simulink model "DFIG_LVRT_function_add_20210713_v1"  (R2021a)
settings: Solver=VariableStepAuto  StartTime=0.0  StopTime=4.3  FixedStep=50e-6  RelTol=1e-3
InitFcn:
  | init;
values from neighbouring files (symbols this model uses):
  a11 = -Rs/sigma/Ls    (= -15.198082107)    [init.m]
  a13 = Rs*Lm/sigma/Ls/Lr    (= 14.6869753643)    [init.m]
  a22 = a11    (= -15.198082107)    [init.m]
  a24 = a13    (= 14.6869753643)    [init.m]
  a31 = Rr*Lm/sigma/Ls/Lr    (= 16.3816263679)    [init.m]
  a33 = -Rr/sigma/Ls    (= -16.9517069655)    [init.m]
  a42 = a31    (= 16.3816263679)    [init.m]
  a44 = a33    (= -16.9517069655)    [init.m]
  Cbus = 80e-3    (= 0.08)    [init.m]
  D = 1e-3 * 0    (= 0)    [init.m]
  f = 50    [init.m]
  Fs = Vs * sqrt(2/3)/(2*pi*f)    [init.m]
  fsw = 4e3    (= 4000)    [init.m]
  Is = 1760    [init.m]
  J = 127    [init.m]
  Kopt = ((0.5*ro*pi*(Rayon^5)*Cp_max)/(lambda_opt^3))    (= 296454.198186)    [init.m]
  Kpg = 1/(1.5*Vs*sqrt(2/3))    [init.m]
  Kqg = -Kpg    [init.m]
  Lg = 400e-6    (= 0.0004)    [init.m]
  Lm = 2.5e-3    (= 0.0025)    [init.m]
  Lr = Lm + Lsi    (= 0.002587)    [init.m]
  Ls = Lm + Lsi    (= 0.002587)    [init.m]
  Lsi = 0.087e-3    (= 8.7e-05)    [init.m]
  N = 100    [init.m]
  p = 2    [init.m]
  Ps = 2e6    (= 2000000)    [init.m]
  Rcrowbar = 1/5    (= 0.2)    [init.m]
  Rg = 20e-6    (= 2e-05)    [init.m]
  Rr = 2.9e-3    (= 0.0029)    [init.m]
  Rs = 2.6e-3    (= 0.0026)    [init.m]
  sigma = 1 - Lm^2/(Ls*Lr)    (= 0.0661284179513)    [init.m]
  smax = 1/3    (= 0.333333333333)    [init.m]
  Tem = 12732    [init.m]
  Ts = 1/fsw/50    (= 5e-06)    [init.m]
  Vbus = 1150    [init.m]
  Vs = 690    [init.m]
undefined symbols (not defined in the file or in its folder): DiscIntNeverNeededParam
libraries: DFIM_Tutorial_Library x37, spsSecondOrderFilterLib x8, spsSeriesRLCBranchLib x5, spsThreePhaseVIMeasurementLib x4, spsUniversalBridgeLib x3, spsPLL3phLib x2, spsPWMGenerator2LevelLib x2, spsAsynchronousMachineSIUnitsLib x1, spsGroundLib x1, spsThreePhaseTransformerTwoWindingsLib x1, spsIdealSwitchLib x1, spsMultimeterLib x1
settings Model: SimulationMode=accelerator  Creator=anony  LastModifiedBy=anony
settings SolverCC: AlgebraicLoopSolver=TrustRegion
settings DebuggingCC: UnconnectedInputMsg=none  UnconnectedOutputMsg=none  UnconnectedLineMsg=none  SFMachineParentedDataDiag=warning

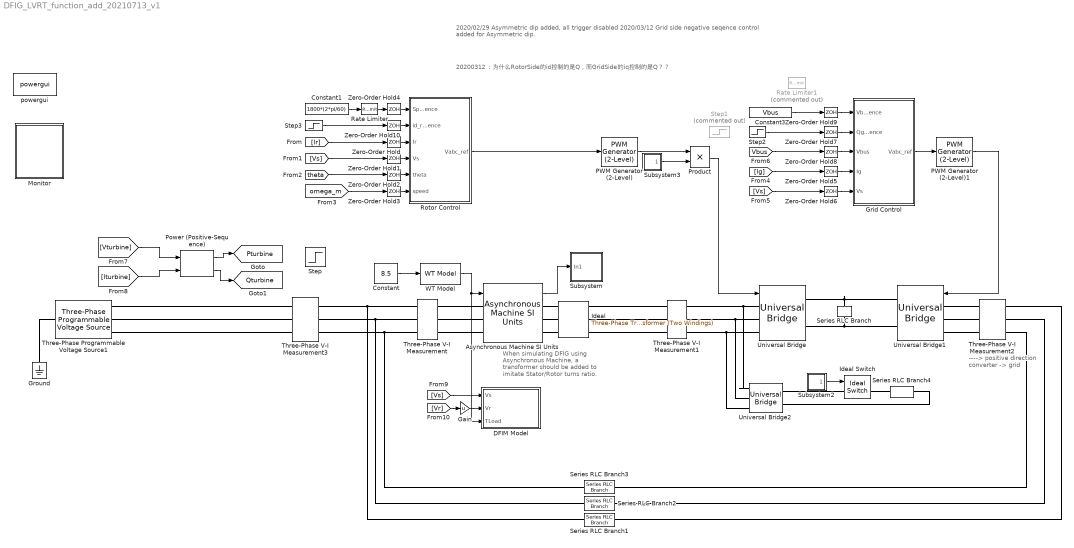
== system DFIG_LVRT_function_add_20210713_v1 ==
  note: 20200312：为什么RotorSide的id控制的是Q，而GridSide的iq控制的是Q？？
  note: ---->
      | positive direction
      | converter -> grid
  note: When simulating DFIG using Asynchronous Machine,
      | a transformer should be added to imitate Stator/Rotor turns
      | ratio.
  note: 2020/02/29 Asymmetric dip added, all trigger disabled
      | 2020/03/12 Grid side negative seqence control added for Asymmetric dip.
  Asynchronous Machine SI Units : spsAsynchronousMachineSIUnitsLib/Asynchronous Machine SI Units  RotorType=Wound  PresetModel=No  MechanicalLoad=Torque Tm  ShowDetailedParameters=on  ReferenceFrame=Rotor  Units=SI  MeasurementBus=off  NominalParameters=[Ps Vs f]  VoltageRatio=1  Stator=[Rs Lsi]  Rotor=[Rr Lsi]  Cage1=[0.4155 0.002066]  Cage2=[0.4168 0.0003495]  Lm=Lm  Mechanical=[J D p]  PolePairs=2  InitialConditions=[1 0 0 0 0 0 0 0]  SimulateSaturation=off  Saturation=[14.03593122, 27.81365428, 53.79336849, 72.68890987, 97.98006896, 148.6815601, 215.7428561, 302.9841135, 428.7778367 ; 230, 322, 414, 460, 506, 552, 598, 644, 690]  LoadFlowParameters=1492000  TsPowergui=0  TsBlock=-1  IterativeModel=Trapezoidal non iterative  IterativeDiscreteModel=Trapezoidal non iterative  Pmec=1.492e+006
  Constant : Constant  Value=8.5
  Constant1 : Constant  Value=1800*(2*pi/60)
  Constant3 : Constant  Value=Vbus
  DFIM Model : Subsystem
  Gain : Gain  Gain=u
  Grid Control : Subsystem
  Ground : spsGroundLib/Ground  LConnTagsString=a
  Ideal : spsThreePhaseTransformerTwoWindingsLib/Three-Phase Transformer (Two Windings)  Winding1Connection=Y  Winding2Connection=Y  CoreType=Three single-phase transformers  SetSaturation=off  Hysteresis=off  DataFile='hysteresis'  SetInitialFlux=off  Measurements=None  UNITS=SI  NominalPower=[ Ps , f ]  Winding1=[Vs 0 0]  Winding2=[Vs/u 0 0]  Rm="1.0805e+06  % keep this at a high value"  Lm="2866  % keep this at a high value"  L0=0.5  Saturation=[0 0;0.66653 1910.3;277.72 2419.7]  InitialFluxes=[ 0.8 , -0.8 , 0.7 ]  BreakLoop=off  DiscreteSolver=Trapezoidal iterative  DataType=on  TransfoNumber=1
  Ideal Switch : spsIdealSwitchLib/Ideal Switch  Ron=0.001  Lon=0  IC=0  Rs=1e5  Cs=inf  Measurements=on
  Monitor : Subsystem
  PWM Generator (2-Level) : spsPWMGenerator2LevelLib/PWM Generator (2-Level)  ModulatorType=Three-phase bridge (6 pulses)  ModulatorMode=Unsynchronized  Fc=fsw  Pc=90  nF=27  MinMax="[ -1  1 ]"  SamplingTechnique=Symmetrical regular (single edge)  ModulatingSignals=off  m=0.8  Freq=60  Phase=0  Ts=0  ShowCarrierOutport=off
  PWM Generator (2-Level)1 : spsPWMGenerator2LevelLib/PWM Generator (2-Level)  ModulatorType=Three-phase bridge (6 pulses)  ModulatorMode=Unsynchronized  Fc=fsw  Pc=0  nF=27  MinMax="[ -1  1 ]"  SamplingTechnique=Symmetrical regular (single edge)  ModulatingSignals=off  m=0.8  Freq=60  Phase=0  Ts=0  ShowCarrierOutport=off
  Power (Positive-Sequence) : spsPowerPositiveSequenceLib/Power (Positive-Sequence)  Freq=50  Vinit=[0, 0]  Iinit=[0, 0]  Ts=0
      settings: SourceProductBaseCode=PS
  Product : Product
  Rate Limiter : RateLimiter  RisingSlewLimit=100/1  FallingSlewLimit=-100/1  SampleTimeMode=inherited
  Rate Limiter1 : RateLimiter  Commented=on  RisingSlewLimit=1000e3/2  FallingSlewLimit=-1000e3/2  SampleTimeMode=inherited
  Rotor Control : Subsystem
  Series RLC Branch : spsSeriesRLCBranchLib/Series RLC Branch  LConnTagsString=__new0  RConnTagsString=__new0  BranchType=C  Resistance=1  Inductance=1e-3  SetiL0=off  InitialCurrent=0  Capacitance=Cbus  Setx0=on  InitialVoltage=0  Measurements=Branch voltage
  Series RLC Branch1 : spsSeriesRLCBranchLib/Series RLC Branch  LConnTagsString=__new0  RConnTagsString=__new0  BranchType=RL  Resistance=Rg  Inductance=Lg  SetiL0=off  InitialCurrent=0  Capacitance=Cbus  Setx0=on  InitialVoltage=0  Measurements=None
  Series RLC Branch2 : spsSeriesRLCBranchLib/Series RLC Branch  LConnTagsString=__new0  RConnTagsString=__new0  BranchType=RL  Resistance=Rg  Inductance=Lg  SetiL0=off  InitialCurrent=0  Capacitance=Cbus  Setx0=on  InitialVoltage=0  Measurements=None
  Series RLC Branch3 : spsSeriesRLCBranchLib/Series RLC Branch  LConnTagsString=__new0  RConnTagsString=__new0  BranchType=RL  Resistance=Rg  Inductance=Lg  SetiL0=off  InitialCurrent=0  Capacitance=Cbus  Setx0=on  InitialVoltage=0  Measurements=None
  Series RLC Branch4 : spsSeriesRLCBranchLib/Series RLC Branch  LConnTagsString=__new0  RConnTagsString=__new0  BranchType=R  Resistance=Rcrowbar  Inductance=1e-3  SetiL0=off  InitialCurrent=0  Capacitance=Cbus  Setx0=on  InitialVoltage=0  Measurements=Branch current
  Step : Step  Time=3.453  Before=7.5  After=11  SampleTime=0
  Step1 : Step  Commented=on  Time=4.084  After=-400e3  SampleTime=0
  Step2 : Step  Time=3.15  After=-500e3  SampleTime=0
  Step3 : Step  Time=3.15  After=Is*0.25  SampleTime=0
  Subsystem : Subsystem
  Subsystem2 : Subsystem
  Subsystem3 : Subsystem
  Three-Phase Programmable Voltage Source1 : spsThreePhaseProgrammableVoltageSourceLib/Three-Phase Programmable Voltage Source  PositiveSequence=[Vs 0 f]  VariationEntity=None  VariationType=Ramp  VariationTypeAlt=Step  VariationStep=0.5  VariationRate=15  VariationMagnitude=0.3  VariationFrequency=2  VariationTiming=[3.5 4.17]  VariationPhaseA=off  Amplitudes=[1 0.8 1.2 1.0]  TimeValues=[0 0.1 0.15 0.2]  HarmonicGeneration=on  HarmonicA=[1 0.3 180 1]  HarmonicB=[1 0.2 0 2]  Timing="[3  4.2]"  BusType=swing  Pref=0  Qref=0  Qmin=-inf  Qmax=inf
  Three-Phase V-I Measurement : spsThreePhaseVIMeasurementLib/Three-Phase V-I Measurement  VoltageMeasurement=phase-to-ground  SetLabelV=on  LabelV=Vs  Vpu=off  VpuLL=off  CurrentMeasurement=yes  SetLabelI=on  LabelI=Is  Ipu=off  Pbase=100e6  Vbase=500e3  OutputType=Complex  PhasorSimulation=off  PSBequivalent=0
  Three-Phase V-I Measurement1 : spsThreePhaseVIMeasurementLib/Three-Phase V-I Measurement  VoltageMeasurement=phase-to-ground  SetLabelV=on  LabelV=Vr  Vpu=off  VpuLL=off  CurrentMeasurement=yes  SetLabelI=on  LabelI=Ir  Ipu=off  Pbase=100e6  Vbase=500e3  OutputType=Complex  PhasorSimulation=off  PSBequivalent=0
  Three-Phase V-I Measurement2 : spsThreePhaseVIMeasurementLib/Three-Phase V-I Measurement  VoltageMeasurement=no  SetLabelV=on  LabelV=Vs  Vpu=on  VpuLL=off  CurrentMeasurement=yes  SetLabelI=on  LabelI=Ig  Ipu=off  Pbase=100e6  Vbase=500e3  OutputType=Complex  PhasorSimulation=off  PSBequivalent=0
  Three-Phase V-I Measurement3 : spsThreePhaseVIMeasurementLib/Three-Phase V-I Measurement  VoltageMeasurement=phase-to-ground  SetLabelV=on  LabelV=Vturbine  Vpu=off  VpuLL=off  CurrentMeasurement=yes  SetLabelI=on  LabelI=Iturbine  Ipu=off  Pbase=100e6  Vbase=500e3  OutputType=Complex  PhasorSimulation=off  PSBequivalent=0
  Universal Bridge : spsUniversalBridgeLib/Universal Bridge  Arms=3  SnubberResistance=1e5  SnubberCapacitance=inf  Device=Ideal Switches  Ron=1e-3  Lon=0  ForwardVoltages="[  0  0  ]"  ForwardVoltage=0  GTOparameters=[ 10e-6 , 20e-6 ]  IGBTparameters=[ 1e-6 , 2e-6 ]  Measurements=None  Measurements_2=None  converterType=Rectifier
  Universal Bridge1 : spsUniversalBridgeLib/Universal Bridge  Arms=3  SnubberResistance=1e5  SnubberCapacitance=inf  Device=Ideal Switches  Ron=1e-3  Lon=0  ForwardVoltages="[  0  0  ]"  ForwardVoltage=0  GTOparameters=[ 10e-6 , 20e-6 ]  IGBTparameters=[ 1e-6 , 2e-6 ]  Measurements=None  Measurements_2=None  converterType=Rectifier
  Universal Bridge2 : spsUniversalBridgeLib/Universal Bridge  Arms=3  SnubberResistance=1e5  SnubberCapacitance=inf  Device=Diodes  Ron=1e-3  Lon=0  ForwardVoltages="[  0  0  ]"  ForwardVoltage=0  GTOparameters=[ 10e-6 , 20e-6 ]  IGBTparameters=[ 1e-6 , 2e-6 ]  Measurements=None  Measurements_2=None  converterType=Rectifier
  WT Model : DFIM_Tutorial_Library/WT Model  SystemSampleTime=-1  VariantActivationTime=update diagram  Latency=0  AutoFrameSizeCalculation=off
  Zero-Order Hold{,1..10} (11 alike) : ZeroOrderHold  SampleTime=1/fsw
  powergui : spspowerguiLib/powergui  Priority=1  SimulationMode=Discrete  SampleTime=Ts  frequency=60  Iterations=50  frequencyindice=50  Pbase=100e6  ErrMax=1e-4  UnitsV=kV  UnitsW=MW  buscounter=0  FunctionMessages=off  echomessages=off  EnableUseOfTLC=off  CurrentSourceSwitches=off  DisableSnubberDevices=off  DisableRonSwitches=off  DisableVfSwitches=off  DisplayEquations=off  AutomaticDiscreteSolvers=off  SolverType=Tustin/Backward Euler (TBE)  Interpol=off  ExternalGateDelay=off  methode=off  Ts=100  x0status=blocks  SPID=on  SwTol=0  HookPort=off  NonlinearTolerance=1e-4  nMaxIteration=100  ContinueOnMaxIteration=off  RestoreLinks=warning  ResistiveCurrentMeasurement=off  Frange=[0:2:500]  Ylog=off  Xlog=on  ShowGrid=off  save=off  variable=ZData  structure=0  ZoomFFT=off  StartTime=0.0  cycles=1  DisplayStyle=1  fundamental=60  FreqAxis=off  MaxFrequency=1000  frequencyindicesteady=1  RmsSteady=1  display=off
  tag scope: Pturbine=global, Qturbine=global
  wires:
  Rotor Control/1(Vabc_ref) -> PWM Generator (2-Level)/1
  [Ir] -> Zero-Order Hold/1
  [Vs] -> Zero-Order Hold1/1
  Asynchronous Machine SI Units/1 -> Subsystem/1(In1)
  [theta] -> Zero-Order Hold2/1
  [omega_m] -> Zero-Order Hold3/1
  Step3/1 -> Zero-Order Hold10/1
  Zero-Order Hold/1 -> Rotor Control/3(Ir)
  Zero-Order Hold1/1 -> Rotor Control/4(Vs)
  Zero-Order Hold2/1 -> Rotor Control/5(theta)
  Zero-Order Hold3/1 -> Rotor Control/6(speed)
  Constant1/1 -> Rate Limiter/1
  Rate Limiter/1 -> Zero-Order Hold4/1
  Zero-Order Hold4/1 -> Rotor Control/1(Speed reference)
  WT Model/1 -> DFIM Model/3(TLoad), Asynchronous Machine SI Units/1
  PWM Generator (2-Level)1/1 -> Universal Bridge1/1
  Zero-Order Hold5/1 -> Grid Control/4(Ig)
  [Vs] -> Zero-Order Hold6/1
  Zero-Order Hold6/1 -> Grid Control/5(Vs)
  [Ig] -> Zero-Order Hold5/1
  Zero-Order Hold9/1 -> Grid Control/1(Vbus reference)
  Constant3/1 -> Zero-Order Hold9/1
  Grid Control/1(Vabc_ref) -> PWM Generator (2-Level)1/1
  Step2/1 -> Zero-Order Hold7/1
  Zero-Order Hold7/1 -> Grid Control/2(Qg_reference)
  [Vbus] -> Zero-Order Hold8/1
  Zero-Order Hold8/1 -> Grid Control/3(Vbus)
  Subsystem2/1(Trig) -> Ideal Switch/1
  Zero-Order Hold10/1 -> Rotor Control/2(id_reference)
  Subsystem3/1(Trig) -> Product/2
  PWM Generator (2-Level)/1 -> Product/1
  Product/1 -> Universal Bridge/1
  Constant/1 -> WT Model/1
  [Vturbine] -> Power (Positive-Sequence)/1
  [Iturbine] -> Power (Positive-Sequence)/2
  Power (Positive-Sequence)/2 -> [Qturbine]
  Power (Positive-Sequence)/1 -> [Pturbine]
  [Vs] -> DFIM Model/1(Vs)
  [Vr] -> Gain/1
  Gain/1 -> DFIM Model/2(Vr)
  connections:
  Three-Phase Programmable Voltage Source1/LConn1 -- Ground/LConn1
  Three-Phase V-I Measurement1/LConn1 -- Universal Bridge2/LConn1 -- Universal Bridge/LConn1
  Three-Phase V-I Measurement1/LConn2 -- Universal Bridge2/LConn2 -- Universal Bridge/LConn2
  Three-Phase V-I Measurement1/LConn3 -- Universal Bridge2/LConn3 -- Universal Bridge/LConn3
  Series RLC Branch1/RConn1 -- Three-Phase V-I Measurement3/LConn1 -- Three-Phase V-I Measurement/LConn1
  Series RLC Branch2/RConn1 -- Three-Phase V-I Measurement/LConn2 -- Three-Phase V-I Measurement3/LConn2
  Series RLC Branch3/RConn1 -- Three-Phase V-I Measurement3/LConn3 -- Three-Phase V-I Measurement/LConn3
  Three-Phase V-I Measurement/RConn1 -- Asynchronous Machine SI Units/LConn1
  Three-Phase V-I Measurement/RConn2 -- Asynchronous Machine SI Units/LConn2
  Three-Phase V-I Measurement/RConn3 -- Asynchronous Machine SI Units/LConn3
  Universal Bridge/RConn1 -- Series RLC Branch/LConn1 -- Universal Bridge1/RConn1
  Universal Bridge/RConn2 -- Series RLC Branch/RConn1 -- Universal Bridge1/RConn2
  Three-Phase V-I Measurement2/LConn1 -- Universal Bridge1/LConn1
  Three-Phase V-I Measurement2/LConn2 -- Universal Bridge1/LConn2
  Three-Phase V-I Measurement2/LConn3 -- Universal Bridge1/LConn3
  Series RLC Branch1/LConn1 -- Three-Phase V-I Measurement2/RConn1
  Three-Phase V-I Measurement2/RConn2 -- Series RLC Branch2/LConn1
  Series RLC Branch3/LConn1 -- Three-Phase V-I Measurement2/RConn3
  Ideal/LConn1 -- Asynchronous Machine SI Units/RConn1
  Ideal/LConn2 -- Asynchronous Machine SI Units/RConn2
  Ideal/LConn3 -- Asynchronous Machine SI Units/RConn3
  Ideal/RConn1 -- Three-Phase V-I Measurement1/RConn1
  Ideal/RConn2 -- Three-Phase V-I Measurement1/RConn2
  Ideal/RConn3 -- Three-Phase V-I Measurement1/RConn3
  Series RLC Branch4/LConn1 -- Ideal Switch/RConn1
  Series RLC Branch4/RConn1 -- Universal Bridge2/RConn2
  Universal Bridge2/RConn1 -- Ideal Switch/LConn1
  Three-Phase Programmable Voltage Source1/RConn1 -- Three-Phase V-I Measurement3/RConn1
  Three-Phase Programmable Voltage Source1/RConn2 -- Three-Phase V-I Measurement3/RConn2
  Three-Phase Programmable Voltage Source1/RConn3 -- Three-Phase V-I Measurement3/RConn3

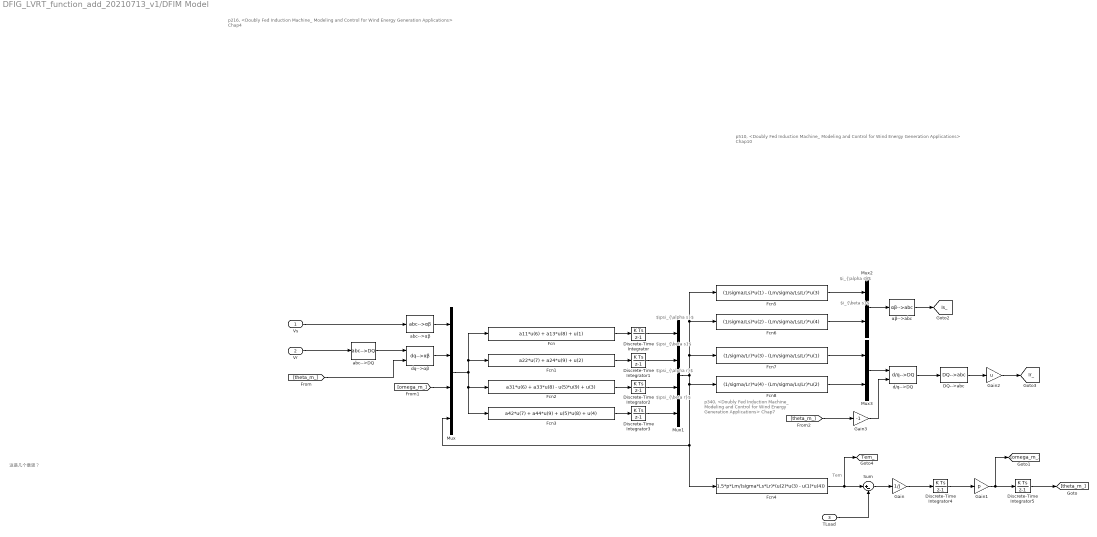
== system DFIG_LVRT_function_add_20210713_v1/DFIM Model ==
  note: p340, <Doubly Fed Induction Machine_ Modeling and Control for Wind Energy Generation Applications> Chap7
  note: $\psi_{\alpha s}$
  note: p510, <Doubly Fed Induction Machine_ Modeling and Control for Wind Energy Generation Applications> Chap10
  note: 这是几个意思？
  note: Tem
  note: p216, <Doubly Fed Induction Machine_ Modeling and Control for Wind Energy Generation Applications> Chap4
  note: $\psi_{\beta s}$
  note: $\psi_{\alpha r}$
  note: $\psi_{\beta r}$
  note: $i_{\alpha s}$
  note: $i_{\beta s}$
  Vs : Inport
  Vr : Inport  Port=2
  TLoad : Inport  Port=3
  DQ-->abc : DFIM_Tutorial_Library/DQ-->abc  SystemSampleTime=-1  VariantActivationTime=update diagram  Latency=0  AutoFrameSizeCalculation=off
  Discrete-Time Integrator{,1..5} (6 alike) : DiscreteIntegrator  SampleTime=Ts  UpperSaturationLimit=1  LowerSaturationLimit=-1  ICPrevOutput=DiscIntNeverNeededParam  ICPrevScaledInput=DiscIntNeverNeededParam
  Fcn : Fcn  Expr=a11*u(6) + a13*u(8) + u(1)
  Fcn1 : Fcn  Expr=a22*u(7) + a24*u(9) + u(2)
  Fcn2 : Fcn  Expr=a31*u(6) + a33*u(8) - u(5)*u(9) + u(3)
  Fcn3 : Fcn  Expr=a42*u(7) + a44*u(9) + u(5)*u(8) + u(4)
  Fcn4 : Fcn  Expr=1.5*p*Lm/(sigma*Ls*Lr)*(u(2)*u(3) - u(1)*u(4))
  Fcn5 : Fcn  Expr=(1/sigma/Ls)*u(1) - (Lm/sigma/Ls/Lr)*u(3)
  Fcn6 : Fcn  Expr=(1/sigma/Ls)*u(2) - (Lm/sigma/Ls/Lr)*u(4)
  Fcn7 : Fcn  Expr=(1/sigma/Lr)*u(3) - (Lm/sigma/Ls/Lr)*u(1)
  Fcn8 : Fcn  Expr=(1/sigma/Lr)*u(4) - (Lm/sigma/Ls/Lr)*u(2)
  Gain : Gain  Gain=1/J
  Gain1 : Gain  Gain=p
  Gain2 : Gain  Gain=u
  Gain3 : Gain  Gain=-1
  Mux : Mux
  Mux1 : Mux
  Mux2 : Mux  Inputs=2
  Mux3 : Mux  Inputs=2
  Sum : Sum  Inputs=|+-
  abc-->DQ : DFIM_Tutorial_Library/abc-->DQ  SystemSampleTime=-1  VariantActivationTime=update diagram  Latency=0  AutoFrameSizeCalculation=off
  abc-->αβ : DFIM_Tutorial_Library/abc-->αβ  SystemSampleTime=-1  VariantActivationTime=update diagram  Latency=0  AutoFrameSizeCalculation=off
  d/q-->DQ : DFIM_Tutorial_Library/d//q-->DQ  SystemSampleTime=-1  VariantActivationTime=update diagram  Latency=0  AutoFrameSizeCalculation=off
  dq-->αβ : DFIM_Tutorial_Library/dq-->αβ  SystemSampleTime=-1  VariantActivationTime=update diagram  Latency=0  AutoFrameSizeCalculation=off
  αβ-->abc : DFIM_Tutorial_Library/αβ-->abc  SystemSampleTime=-1  VariantActivationTime=update diagram  Latency=0  AutoFrameSizeCalculation=off
  tag scope: Ir_=global, Is_=global, Tem_=global
  wires:
  Mux/1 -> Fcn3/1, Fcn2/1, Fcn1/1, Fcn/1
  Fcn/1 -> Discrete-Time Integrator/1
  Fcn1/1 -> Discrete-Time Integrator1/1
  Fcn2/1 -> Discrete-Time Integrator2/1
  Fcn3/1 -> Discrete-Time Integrator3/1
  Discrete-Time Integrator1/1 -> Mux1/2
  Discrete-Time Integrator/1 -> Mux1/1
  Discrete-Time Integrator2/1 -> Mux1/3
  Discrete-Time Integrator3/1 -> Mux1/4
  Mux1/1 -> Fcn7/1, Fcn6/1, Fcn5/1, Mux/4, Fcn4/1, Fcn8/1
  Gain/1 -> Discrete-Time Integrator4/1
  Discrete-Time Integrator4/1 -> Gain1/1
  Gain1/1 -> [omega_m_], Discrete-Time Integrator5/1
  Discrete-Time Integrator5/1 -> [theta_m_]
  Sum/1 -> Gain/1
  Fcn4/1 -> [Tem_], Sum/1
  Vs/1 -> abc-->αβ/1
  abc-->αβ/1 -> Mux/1
  abc-->DQ/1 -> dq-->αβ/1
  dq-->αβ/1 -> Mux/2
  [theta_m_] -> dq-->αβ/2
  Vr/1 -> abc-->DQ/1
  [omega_m_] -> Mux/3
  TLoad/1 -> Sum/2
  Fcn6/1 -> Mux2/2
  Fcn5/1 -> Mux2/1
  Mux2/1 -> αβ-->abc/1
  αβ-->abc/1 -> [Is_]
  DQ-->abc/1 -> Gain2/1
  d/q-->DQ/1 -> DQ-->abc/1
  Fcn7/1 -> Mux3/1
  Fcn8/1 -> Mux3/2
  Gain3/1 -> d/q-->DQ/2
  Mux3/1 -> d/q-->DQ/1
  [theta_m_] -> Gain3/1
  Gain2/1 -> [Ir_]

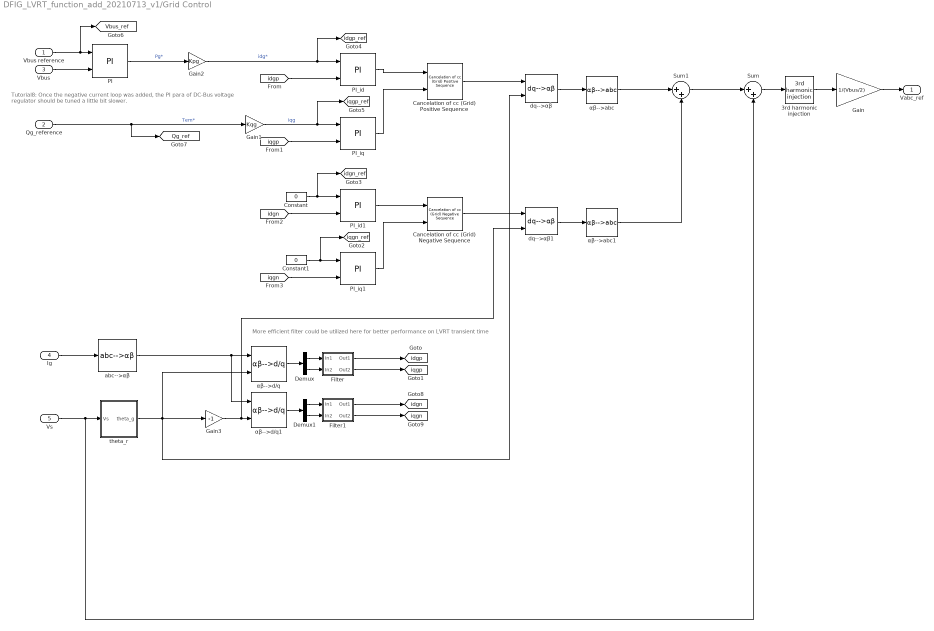
== system DFIG_LVRT_function_add_20210713_v1/Grid Control ==
  note: More efficient filter could be utilized here for better performance on LVRT transient time
  note: Tutorial8: Once the negative current loop was added, the PI para of DC-Bus voltage
      | regulator should be tuned a little bit slower.
  Vbus reference : Inport
  Qg_reference : Inport  Port=2
  Vbus : Inport  Port=3
  Ig : Inport  Port=4
  Vs : Inport  Port=5
  3rd harmonic injection : DFIM_Tutorial_Library/3rd harmonic injection  SystemSampleTime=-1  VariantActivationTime=update diagram  Latency=0  AutoFrameSizeCalculation=off
  Cancelation of cc (Grid) Negative Sequence : DFIM_Tutorial_Library/Cancelation of cc (Grid) Negative Sequence  SystemSampleTime=-1  VariantActivationTime=update diagram  Latency=0  AutoFrameSizeCalculation=off
  Cancelation of cc (Grid) Positive Sequence : DFIM_Tutorial_Library/Cancelation of cc (Grid) Positive Sequence  SystemSampleTime=-1  VariantActivationTime=update diagram  Latency=0  AutoFrameSizeCalculation=off
  Constant : Constant  Value=0
  Constant1 : Constant  Value=0
  Demux : Demux  Outputs=2
  Demux1 : Demux  Outputs=2
  Filter : Subsystem
  Filter1 : Subsystem
  Gain : Gain  Gain=1/(Vbus/2)
  Gain1 : Gain  Gain=Kqg
  Gain2 : Gain  Gain=Kpg
  Gain3 : Gain  Gain=-1
  PI : DFIM_Tutorial_Library/PI  kp=kp_v  ki=ki_v  int_uppper_limit=Ps*smax  int_lower_limit=-Ps*smax  total_upper_limit=Ps*smax  total_lower_limit=-Ps*smax  sample_time=1/fsw
  PI_id : DFIM_Tutorial_Library/PI  kp=kp_idg  ki=ki_idg  int_uppper_limit=Vbus/sqrt(3)  int_lower_limit=-Vbus/sqrt(3)  total_upper_limit=Vbus/sqrt(3)  total_lower_limit=-Vbus/sqrt(3)  sample_time=1/fsw
  PI_id1 : DFIM_Tutorial_Library/PI  kp=kp_idg  ki=ki_idg  int_uppper_limit=Vbus/sqrt(3)  int_lower_limit=-Vbus/sqrt(3)  total_upper_limit=Vbus/sqrt(3)  total_lower_limit=-Vbus/sqrt(3)  sample_time=1/fsw
  PI_iq : DFIM_Tutorial_Library/PI  kp=kp_iqg  ki=ki_iqg  int_uppper_limit=Vbus/sqrt(3)  int_lower_limit=-Vbus/sqrt(3)  total_upper_limit=Vbus/sqrt(3)  total_lower_limit=-Vbus/sqrt(3)  sample_time=1/fsw
  PI_iq1 : DFIM_Tutorial_Library/PI  kp=kp_iqg  ki=ki_iqg  int_uppper_limit=Vbus/sqrt(3)  int_lower_limit=-Vbus/sqrt(3)  total_upper_limit=Vbus/sqrt(3)  total_lower_limit=-Vbus/sqrt(3)  sample_time=1/fsw
  Sum : Sum  Inputs=|++
  Sum1 : Sum  Inputs=|++
  abc-->αβ : DFIM_Tutorial_Library/abc-->αβ  SystemSampleTime=-1  VariantActivationTime=update diagram  Latency=0  AutoFrameSizeCalculation=off
  dq-->αβ : DFIM_Tutorial_Library/dq-->αβ  SystemSampleTime=-1  VariantActivationTime=update diagram  Latency=0  AutoFrameSizeCalculation=off
  dq-->αβ1 : DFIM_Tutorial_Library/dq-->αβ  SystemSampleTime=-1  VariantActivationTime=update diagram  Latency=0  AutoFrameSizeCalculation=off
  theta_r : Subsystem
  αβ-->abc : DFIM_Tutorial_Library/αβ-->abc  SystemSampleTime=-1  VariantActivationTime=update diagram  Latency=0  AutoFrameSizeCalculation=off
  αβ-->abc1 : DFIM_Tutorial_Library/αβ-->abc  SystemSampleTime=-1  VariantActivationTime=update diagram  Latency=0  AutoFrameSizeCalculation=off
  αβ-->d/q : DFIM_Tutorial_Library/αβ-->d//q  SystemSampleTime=-1  VariantActivationTime=update diagram  Latency=0  AutoFrameSizeCalculation=off
  αβ-->d/q1 : DFIM_Tutorial_Library/αβ-->d//q  SystemSampleTime=-1  VariantActivationTime=update diagram  Latency=0  AutoFrameSizeCalculation=off
  Vabc_ref : Outport
  tag scope: Qg_ref=global, Vbus_ref=global, idgn=global, idgn_ref=global, idgp=global, idgp_ref=global, iqgn=global, iqgn_ref=global, iqgp=global, iqgp_ref=global
  wires:
  Gain/1 -> Vabc_ref/1
  dq-->αβ/1 -> αβ-->abc/1
  abc-->αβ/1 -> αβ-->d/q1/1, αβ-->d/q/1
  Ig/1 -> abc-->αβ/1
  3rd harmonic injection/1 -> Gain/1
  Vs/1 -> Sum/2, theta_r/1(Vs)
  theta_r/1(theta_g) -> αβ-->d/q/2, dq-->αβ/2, Gain3/1
  PI_id/1 -> Cancelation of cc (Grid) Positive Sequence/1
  Cancelation of cc (Grid) Positive Sequence/1 -> dq-->αβ/1
  PI_iq/1 -> Cancelation of cc (Grid) Positive Sequence/2
  αβ-->d/q/1 -> Demux/1
  Vbus reference/1 -> [Vbus_ref], PI/1
  Gain1/1 -> [iqgp_ref], PI_iq/1  "iqg"
  Qg_reference/1 -> [Qg_ref], Gain1/1  "Tem*"
  PI/1 -> Gain2/1  "Pg*"
  Gain2/1 -> [idgp_ref], PI_id/1  "idg*"
  Vbus/1 -> PI/2
  Sum/1 -> 3rd harmonic injection/1
  dq-->αβ1/1 -> αβ-->abc1/1
  PI_id1/1 -> Cancelation of cc (Grid) Negative Sequence/1
  Cancelation of cc (Grid) Negative Sequence/1 -> dq-->αβ1/1
  PI_iq1/1 -> Cancelation of cc (Grid) Negative Sequence/2
  αβ-->abc/1 -> Sum1/1
  Sum1/1 -> Sum/1
  αβ-->abc1/1 -> Sum1/2
  Constant/1 -> [idgn_ref], PI_id1/1
  Constant1/1 -> [iqgn_ref], PI_iq1/1
  Demux/1 -> Filter/1(In1)
  Demux/2 -> Filter/2(In2)
  Filter/1(Out1) -> [idgp]
  Filter/2(Out2) -> [iqgp]
  Filter1/2(Out2) -> [iqgn]
  Filter1/1(Out1) -> [idgn]
  Demux1/2 -> Filter1/2(In2)
  Demux1/1 -> Filter1/1(In1)
  αβ-->d/q1/1 -> Demux1/1
  Gain3/1 -> dq-->αβ1/2, αβ-->d/q1/2
  [idgp] -> PI_id/2
  [iqgp] -> PI_iq/2
  [iqgn] -> PI_iq1/2
  [idgn] -> PI_id1/2

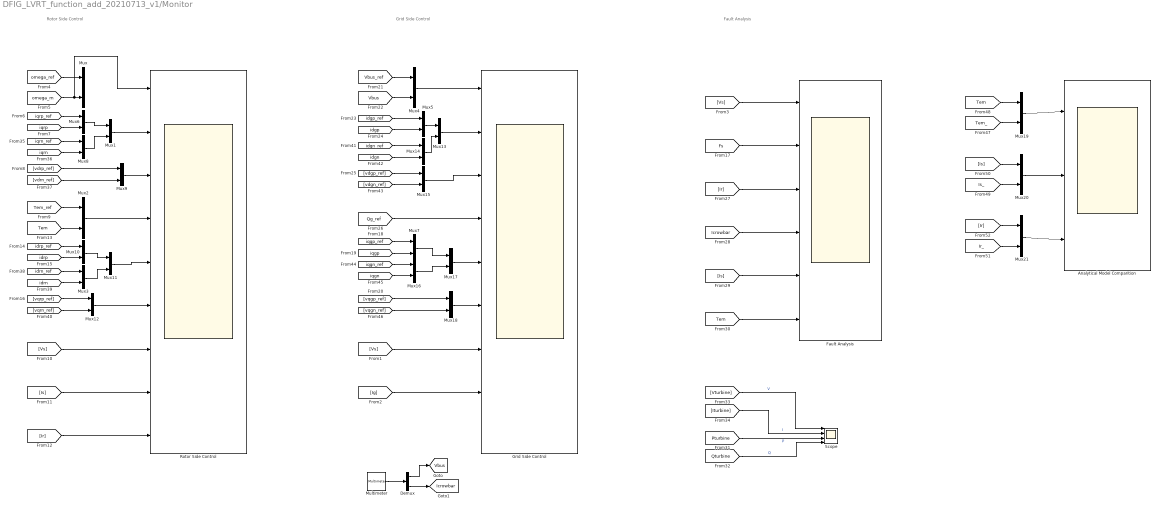
== system DFIG_LVRT_function_add_20210713_v1/Monitor ==
  note: Rotor Side Control
  note: Grid Side Control
  note: Fault Analysis
  Analytical Model Comparition : Scope  NumInputPorts=3
  Demux : Demux  Outputs=2
  Fault Analysis : Scope  NumInputPorts=6
  Grid Side Control : Scope  NumInputPorts=9
  Multimeter : spsMultimeterLib/Multimeter  PhasorSimulation=off  OutputType=Complex  sel=[1 2]  L=2  Gain=[1 1]  yselected={'Ub: Series RLC Branch','Ib: Series RLC Branch4'};  PSBOutputType=1  PSBequivalent=0  AxesSetting=[0,0.1,-100,100]  Display=0  SavedBlockNames=-11
  Mux{,1..21} (22 alike) : Mux  Inputs=2
  Rotor Side Control : Scope  NumInputPorts=9
  Scope : Scope  NumInputPorts=4
  tag scope: Icrowbar=global, Vbus=global
  wires:
  [Tem_ref] -> Mux2/1
  [Ir] -> Rotor Side Control/9
  [Vs] -> Rotor Side Control/7
  [iqrp_ref] -> Mux6/1
  [Tem] -> Mux2/2
  [iqrp] -> Mux6/2
  Mux2/1 -> Rotor Side Control/4
  [Is] -> Rotor Side Control/8
  [omega_m] -> Rotor Side Control/1, Mux/2
  [omega_ref] -> Mux/1
  [Vbus_ref] -> Mux4/1
  [Vbus] -> Mux4/2
  [iqgp_ref] -> Mux7/1
  [Ig] -> Grid Side Control/8
  [idgp] -> Mux5/2
  [iqgp] -> Mux7/2
  [idgp_ref] -> Mux5/1
  [Vs] -> Grid Side Control/7
  [Qg_ref] -> Grid Side Control/4
  Mux4/1 -> Grid Side Control/1
  Multimeter/1 -> Demux/1
  Demux/1 -> [Vbus]
  Demux/2 -> [Icrowbar]
  [Vs] -> Fault Analysis/1
  [Fs] -> Fault Analysis/2
  [Ir] -> Fault Analysis/3
  [Icrowbar] -> Fault Analysis/4
  [Is] -> Fault Analysis/5
  [Tem] -> Fault Analysis/6
  [Pturbine] -> Scope/3  "P"
  [Qturbine] -> Scope/4  "Q"
  [Iturbine] -> Scope/2  "I"
  [Vturbine] -> Scope/1  "V"
  [iqrn_ref] -> Mux8/1
  [iqrn] -> Mux8/2
  Mux6/1 -> Mux1/1
  Mux8/1 -> Mux1/2
  Mux1/1 -> Rotor Side Control/2
  Mux9/1 -> Rotor Side Control/3
  [vdrp_ref] -> Mux9/1
  [vdrn_ref] -> Mux9/2
  [idrp_ref] -> Mux10/1
  [idrp] -> Mux10/2
  [idrn_ref] -> Mux3/1
  [idrn] -> Mux3/2
  Mux10/1 -> Mux11/1
  Mux3/1 -> Mux11/2
  Mux11/1 -> Rotor Side Control/5
  Mux12/1 -> Rotor Side Control/6
  [vqrp_ref] -> Mux12/1
  [vqrn_ref] -> Mux12/2
  Mux13/1 -> Grid Side Control/2
  Mux5/1 -> Mux13/1
  [idgn_ref] -> Mux14/1
  [idgn] -> Mux14/2
  Mux14/1 -> Mux13/2
  Mux15/1 -> Grid Side Control/3
  [vdgp_ref] -> Mux15/1
  [vdgn_ref] -> Mux15/2
  [iqgn] -> Mux16/2
  [iqgn_ref] -> Mux16/1
  Mux17/1 -> Grid Side Control/5
  Mux7/1 -> Mux17/1
  Mux16/1 -> Mux17/2
  Mux18/1 -> Grid Side Control/6
  [vqgp_ref] -> Mux18/1
  [vqgn_ref] -> Mux18/2
  [Tem] -> Mux19/1
  [Tem_] -> Mux19/2
  [Is_] -> Mux20/2
  [Is] -> Mux20/1
  [Ir] -> Mux21/1
  [Ir_] -> Mux21/2
  Mux19/1 -> Analytical Model Comparition/1
  Mux20/1 -> Analytical Model Comparition/2
  Mux21/1 -> Analytical Model Comparition/3

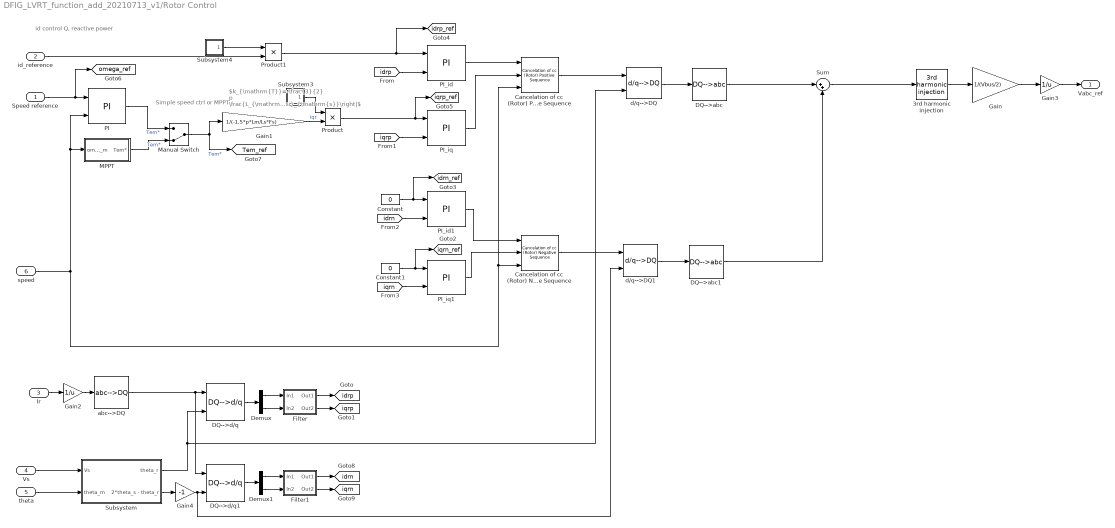
== system DFIG_LVRT_function_add_20210713_v1/Rotor Control ==
  note: id control Q, reactive power
  note: Simple speed ctrl
      | or MPPT
  note: $k_{\mathrm{T}}=-\frac{3}{2} p \frac{L_{\mathrm{m}}}{L_{\mathrm{s}}}\left|\bar{\psi}_{\mathrm{s}}\right|$
  Speed reference : Inport
  id_reference : Inport  Port=2
  Ir : Inport  Port=3
  Vs : Inport  Port=4
  theta : Inport  Port=5
  speed : Inport  Port=6
  3rd harmonic injection : DFIM_Tutorial_Library/3rd harmonic injection  SystemSampleTime=-1  VariantActivationTime=update diagram  Latency=0  AutoFrameSizeCalculation=off
  Cancelation of cc (Rotor) Negative Sequence : DFIM_Tutorial_Library/Cancelation of cc (Rotor) Negative Sequence  SystemSampleTime=-1  VariantActivationTime=update diagram  Latency=0  AutoFrameSizeCalculation=off
  Cancelation of cc (Rotor) Positive Sequence : DFIM_Tutorial_Library/Cancelation of cc (Rotor) Positive Sequence  SystemSampleTime=-1  VariantActivationTime=update diagram  Latency=0  AutoFrameSizeCalculation=off
  Constant : Constant  Value=0
  Constant1 : Constant  Value=0
  DQ-->abc : DFIM_Tutorial_Library/DQ-->abc  SystemSampleTime=-1  VariantActivationTime=update diagram  Latency=0  AutoFrameSizeCalculation=off
  DQ-->abc1 : DFIM_Tutorial_Library/DQ-->abc  SystemSampleTime=-1  VariantActivationTime=update diagram  Latency=0  AutoFrameSizeCalculation=off
  DQ-->d/q : DFIM_Tutorial_Library/DQ-->d//q  SystemSampleTime=-1  VariantActivationTime=update diagram  Latency=0  AutoFrameSizeCalculation=off
  DQ-->d/q1 : DFIM_Tutorial_Library/DQ-->d//q  SystemSampleTime=-1  VariantActivationTime=update diagram  Latency=0  AutoFrameSizeCalculation=off
  Demux : Demux  Outputs=2
  Demux1 : Demux  Outputs=2
  Filter : Subsystem
  Filter1 : Subsystem
  Gain : Gain  Gain=1/(Vbus/2)
  Gain1 : Gain  Gain=1/(-1.5*p*Lm/Ls*Fs)
  Gain2 : Gain  Gain=1/u
  Gain3 : Gain  Gain=1/u
  Gain4 : Gain  Gain=-1
  MPPT : Subsystem
  Manual Switch : ManualSwitch  CurrentSetting=0
  PI : DFIM_Tutorial_Library/PI  kp=kp_n  ki=ki_n  int_uppper_limit=Tem  int_lower_limit=-Tem  total_upper_limit=Tem  total_lower_limit=-Tem  sample_time=1/fsw
  PI_id : DFIM_Tutorial_Library/PI  kp=kp_id  ki=ki_id  int_uppper_limit=Vbus/sqrt(3)  int_lower_limit=-Vbus/sqrt(3)  total_upper_limit=Vbus/sqrt(3)  total_lower_limit=-Vbus/sqrt(3)  sample_time=1/fsw
  PI_id1 : DFIM_Tutorial_Library/PI  kp=kp_id  ki=ki_id  int_uppper_limit=Vbus/sqrt(3)  int_lower_limit=-Vbus/sqrt(3)  total_upper_limit=Vbus/sqrt(3)  total_lower_limit=-Vbus/sqrt(3)  sample_time=1/fsw
  PI_iq : DFIM_Tutorial_Library/PI  kp=kp_iq  ki=ki_iq  int_uppper_limit=Vbus/sqrt(3)  int_lower_limit=-Vbus/sqrt(3)  total_upper_limit=Vbus/sqrt(3)  total_lower_limit=-Vbus/sqrt(3)  sample_time=1/fsw
  PI_iq1 : DFIM_Tutorial_Library/PI  kp=kp_iq  ki=ki_iq  int_uppper_limit=Vbus/sqrt(3)  int_lower_limit=-Vbus/sqrt(3)  total_upper_limit=Vbus/sqrt(3)  total_lower_limit=-Vbus/sqrt(3)  sample_time=1/fsw
  Product : Product
  Product1 : Product
  Subsystem : Subsystem
  Subsystem3 : Subsystem
  Subsystem4 : Subsystem
  Sum : Sum  Inputs=|++
  abc-->DQ : DFIM_Tutorial_Library/abc-->DQ  SystemSampleTime=-1  VariantActivationTime=update diagram  Latency=0  AutoFrameSizeCalculation=off
  d/q-->DQ : DFIM_Tutorial_Library/d//q-->DQ  SystemSampleTime=-1  VariantActivationTime=update diagram  Latency=0  AutoFrameSizeCalculation=off
  d/q-->DQ1 : DFIM_Tutorial_Library/d//q-->DQ  SystemSampleTime=-1  VariantActivationTime=update diagram  Latency=0  AutoFrameSizeCalculation=off
  Vabc_ref : Outport
  tag scope: Tem_ref=global, idrn=global, idrn_ref=global, idrp=global, idrp_ref=global, iqrn=global, iqrn_ref=global, iqrp=global, iqrp_ref=global, omega_ref=global
  wires:
  Gain/1 -> Gain3/1
  d/q-->DQ/1 -> DQ-->abc/1
  abc-->DQ/1 -> DQ-->d/q1/1, DQ-->d/q/1
  Ir/1 -> Gain2/1
  3rd harmonic injection/1 -> Gain/1
  Vs/1 -> Subsystem/1(Vs)
  theta/1 -> Subsystem/2(theta_m)
  Subsystem/1(theta_r) -> DQ-->d/q/2, d/q-->DQ/2
  PI_id/1 -> Cancelation of cc (Rotor) Positive Sequence/1
  Cancelation of cc (Rotor) Positive Sequence/1 -> d/q-->DQ/1
  PI_iq/1 -> Cancelation of cc (Rotor) Positive Sequence/2
  speed/1 -> MPPT/1(omega_m), PI/2, Cancelation of cc (Rotor) Positive Sequence/3, Cancelation of cc (Rotor) Negative Sequence/3
  DQ-->d/q/1 -> Demux/1
  Speed reference/1 -> [omega_ref], PI/1
  Manual Switch/1 -> Gain1/1, [Tem_ref]  "Tem*"
  PI/1 -> Manual Switch/1  "Tem*"
  MPPT/1(Tem*) -> Manual Switch/2  "Tem*"
  Gain2/1 -> abc-->DQ/1
  Gain3/1 -> Vabc_ref/1
  Subsystem3/1(Trig) -> Product/1
  Gain1/1 -> Product/2  "iqr"
  Product/1 -> [iqrp_ref], PI_iq/1
  id_reference/1 -> Product1/2
  Product1/1 -> [idrp_ref], PI_id/1
  Subsystem4/1(Trig) -> Product1/1
  DQ-->abc/1 -> Sum/1
  Sum/1 -> 3rd harmonic injection/1
  PI_id1/1 -> Cancelation of cc (Rotor) Negative Sequence/1
  d/q-->DQ1/1 -> DQ-->abc1/1
  Cancelation of cc (Rotor) Negative Sequence/1 -> d/q-->DQ1/1
  Constant/1 -> [idrn_ref], PI_id1/1
  Constant1/1 -> [iqrn_ref], PI_iq1/1
  DQ-->abc1/1 -> Sum/2
  DQ-->d/q1/1 -> Demux1/1
  Subsystem/2(2*theta_s - theta_r) -> Gain4/1
  Gain4/1 -> d/q-->DQ1/2, DQ-->d/q1/2
  Demux/1 -> Filter/1(In1)
  Demux/2 -> Filter/2(In2)
  Filter/1(Out1) -> [idrp]
  Filter/2(Out2) -> [iqrp]
  Demux1/1 -> Filter1/1(In1)
  Demux1/2 -> Filter1/2(In2)
  Filter1/1(Out1) -> [idrn]
  Filter1/2(Out2) -> [iqrn]
  [idrp] -> PI_id/2
  [iqrp] -> PI_iq/2
  [idrn] -> PI_id1/2
  [iqrn] -> PI_iq1/2
  PI_iq1/1 -> Cancelation of cc (Rotor) Negative Sequence/2

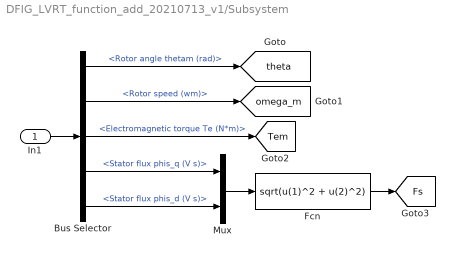
== system DFIG_LVRT_function_add_20210713_v1/Subsystem ==
  In1 : Inport
  Bus Selector : BusSelector  OutputSignals=Mechanical.Rotor angle thetam (rad),Mechanical.Rotor speed (wm),Mechanical.Electromagnetic torque Te (N*m),Stator measurements.Stator flux phis_q (V s),Stator measurements.Stator flux phis_d (V s)
  Fcn : Fcn  Expr=sqrt(u(1)^2 + u(2)^2)
  Mux : Mux  Inputs=2
  tag scope: Fs=global, Tem=global, omega_m=global, theta=global
  wires:
  In1/1 -> Bus Selector/1
  Bus Selector/1 -> [theta]  "<Rotor angle thetam (rad)>"
  Bus Selector/2 -> [omega_m]  "<Rotor speed (wm)>"
  Bus Selector/3 -> [Tem]  "<Electromagnetic torque Te (N*m)>"
  Bus Selector/4 -> Mux/1  "<Stator flux phis_q (V s)>"
  Bus Selector/5 -> Mux/2  "<Stator flux phis_d (V s)>"
  Mux/1 -> Fcn/1
  Fcn/1 -> [Fs]

== system DFIG_LVRT_function_add_20210713_v1/Subsystem2 ==
  Step1 : Step  Time=30.1  After=-1  SampleTime=0
  Step2 : Step  Time=30  SampleTime=0
  Sum : Sum  Inputs=|++
  Trig : Outport
  wires:
  Step2/1 -> Sum/1
  Step1/1 -> Sum/2
  Sum/1 -> Trig/1

== system DFIG_LVRT_function_add_20210713_v1/Subsystem3 ==
  Step1 : Step  Time=30.1  SampleTime=0
  Step2 : Step  Time=30  Before=1  After=0  SampleTime=0
  Sum : Sum  Inputs=|++
  Trig : Outport
  wires:
  Step2/1 -> Sum/1
  Step1/1 -> Sum/2
  Sum/1 -> Trig/1

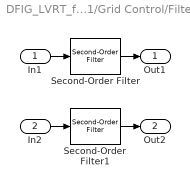
== system DFIG_LVRT_function_add_20210713_v1/Grid Control/Filter ==
  In1 : Inport
  In2 : Inport  Port=2
  Second-Order Filter : spsSecondOrderFilterLib/Second-Order Filter  FilterType=Bandstop (Notch)  Fo=100  Zeta=0.05  Ts=1/fsw  Initialize=off  Vac_Init="[0,  0,  60]"  Vdc_Init=0  PlotResponse=off  FreqRange=[0, 500, 1]
      settings: SourceProductBaseCode=PS
  Second-Order Filter1 : spsSecondOrderFilterLib/Second-Order Filter  FilterType=Bandstop (Notch)  Fo=100  Zeta=0.05  Ts=1/fsw  Initialize=off  Vac_Init="[0,  0,  60]"  Vdc_Init=0  PlotResponse=off  FreqRange=[0, 500, 1]
      settings: SourceProductBaseCode=PS
  Out1 : Outport
  Out2 : Outport  Port=2
  wires:
  Second-Order Filter/1 -> Out1/1
  In1/1 -> Second-Order Filter/1
  In2/1 -> Second-Order Filter1/1
  Second-Order Filter1/1 -> Out2/1

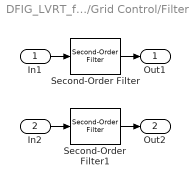
== system DFIG_LVRT_function_add_20210713_v1/Grid Control/Filter1 ==
  In1 : Inport
  In2 : Inport  Port=2
  Second-Order Filter : spsSecondOrderFilterLib/Second-Order Filter  FilterType=Bandstop (Notch)  Fo=100  Zeta=0.05  Ts=1/fsw  Initialize=off  Vac_Init="[0,  0,  60]"  Vdc_Init=0  PlotResponse=off  FreqRange=[0, 500, 1]
      settings: SourceProductBaseCode=PS
  Second-Order Filter1 : spsSecondOrderFilterLib/Second-Order Filter  FilterType=Bandstop (Notch)  Fo=100  Zeta=0.05  Ts=1/fsw  Initialize=off  Vac_Init="[0,  0,  60]"  Vdc_Init=0  PlotResponse=off  FreqRange=[0, 500, 1]
      settings: SourceProductBaseCode=PS
  Out1 : Outport
  Out2 : Outport  Port=2
  wires:
  Second-Order Filter1/1 -> Out2/1
  In2/1 -> Second-Order Filter1/1
  In1/1 -> Second-Order Filter/1
  Second-Order Filter/1 -> Out1/1

== system DFIG_LVRT_function_add_20210713_v1/Grid Control/theta_r ==
  note: Atan2 is used in this version instead of PLL
  note: theta_g
  Vs : Inport
  Constant : Constant  Value=pi/2
  PLL (3ph) : spsPLL3phLib/PLL (3ph)  Fmin=45  Par_Init=[0, 60]  ParK=[180, 3200, 1]  TcD=0.01  MaxRateChangeFreq=12  FilterCutOffFreq=25  Ts=1/fsw  AGC=on
  Sum : Sum  Inputs=|+-
  theta_g : Outport
  wires:
  Constant/1 -> Sum/2
  PLL (3ph)/2 -> Sum/1
  Sum/1 -> theta_g/1
  Vs/1 -> PLL (3ph)/1

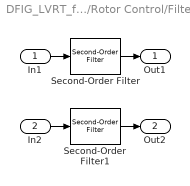
== system DFIG_LVRT_function_add_20210713_v1/Rotor Control/Filter ==
  In1 : Inport
  In2 : Inport  Port=2
  Second-Order Filter : spsSecondOrderFilterLib/Second-Order Filter  FilterType=Bandstop (Notch)  Fo=100  Zeta=0.05  Ts=1/fsw  Initialize=off  Vac_Init="[0,  0,  60]"  Vdc_Init=0  PlotResponse=off  FreqRange=[0, 500, 1]
      settings: SourceProductBaseCode=PS
  Second-Order Filter1 : spsSecondOrderFilterLib/Second-Order Filter  FilterType=Bandstop (Notch)  Fo=100  Zeta=0.05  Ts=1/fsw  Initialize=off  Vac_Init="[0,  0,  60]"  Vdc_Init=0  PlotResponse=off  FreqRange=[0, 500, 1]
      settings: SourceProductBaseCode=PS
  Out1 : Outport
  Out2 : Outport  Port=2
  wires:
  Second-Order Filter/1 -> Out1/1
  In1/1 -> Second-Order Filter/1
  In2/1 -> Second-Order Filter1/1
  Second-Order Filter1/1 -> Out2/1

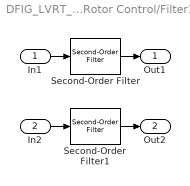
== system DFIG_LVRT_function_add_20210713_v1/Rotor Control/Filter1 ==
  In1 : Inport
  In2 : Inport  Port=2
  Second-Order Filter : spsSecondOrderFilterLib/Second-Order Filter  FilterType=Bandstop (Notch)  Fo=100  Zeta=0.05  Ts=1/fsw  Initialize=off  Vac_Init="[0,  0,  60]"  Vdc_Init=0  PlotResponse=off  FreqRange=[0, 500, 1]
      settings: SourceProductBaseCode=PS
  Second-Order Filter1 : spsSecondOrderFilterLib/Second-Order Filter  FilterType=Bandstop (Notch)  Fo=100  Zeta=0.05  Ts=1/fsw  Initialize=off  Vac_Init="[0,  0,  60]"  Vdc_Init=0  PlotResponse=off  FreqRange=[0, 500, 1]
      settings: SourceProductBaseCode=PS
  Out1 : Outport
  Out2 : Outport  Port=2
  wires:
  Second-Order Filter/1 -> Out1/1
  In1/1 -> Second-Order Filter/1
  In2/1 -> Second-Order Filter1/1
  Second-Order Filter1/1 -> Out2/1

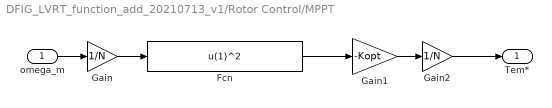
== system DFIG_LVRT_function_add_20210713_v1/Rotor Control/MPPT ==
  omega_m : Inport
  Fcn : Fcn  Expr=u(1)^2
  Gain : Gain  Gain=1/N
  Gain1 : Gain  Gain=-Kopt
  Gain2 : Gain  Gain=1/N
  Tem* : Outport
  wires:
  omega_m/1 -> Gain/1
  Fcn/1 -> Gain1/1
  Gain/1 -> Fcn/1
  Gain1/1 -> Gain2/1
  Gain2/1 -> Tem*/1

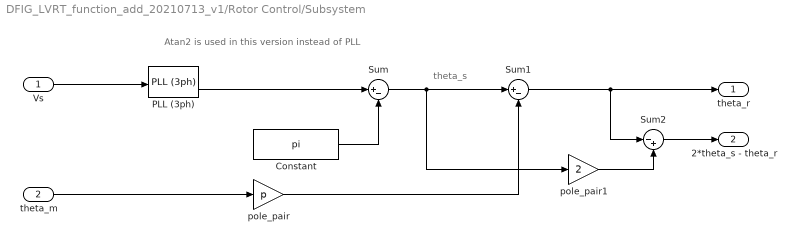
== system DFIG_LVRT_function_add_20210713_v1/Rotor Control/Subsystem ==
  note: Atan2 is used in this version instead of PLL
  note: theta_s
  Vs : Inport
  theta_m : Inport  Port=2
  Constant : Constant  Value=pi
  PLL (3ph) : spsPLL3phLib/PLL (3ph)  Fmin=45  Par_Init=[0, 60]  ParK=[180, 3200, 1]  TcD=0.01  MaxRateChangeFreq=12  FilterCutOffFreq=25  Ts=1/fsw  AGC=on
  Sum : Sum  Inputs=|+-
  Sum1 : Sum  Inputs=|+-
  Sum2 : Sum  Inputs=|-+
  pole_pair : Gain  Gain=p
  pole_pair1 : Gain  Gain=2
  theta_r : Outport
  2*theta_s - theta_r : Outport  Port=2
  wires:
  Vs/1 -> PLL (3ph)/1
  PLL (3ph)/2 -> Sum/1
  Constant/1 -> Sum/2
  Sum/1 -> pole_pair1/1, Sum1/1
  theta_m/1 -> pole_pair/1
  Sum1/1 -> Sum2/1, theta_r/1
  pole_pair/1 -> Sum1/2
  pole_pair1/1 -> Sum2/2
  Sum2/1 -> 2*theta_s - theta_r/1

== system DFIG_LVRT_function_add_20210713_v1/Rotor Control/Subsystem3 ==
  Step1 : Step  Time=40.17  SampleTime=0
  Step2 : Step  Time=30.15  Before=1  After=0  SampleTime=0
  Sum : Sum  Inputs=|++
  Trig : Outport
  wires:
  Sum/1 -> Trig/1
  Step1/1 -> Sum/2
  Step2/1 -> Sum/1

== system DFIG_LVRT_function_add_20210713_v1/Rotor Control/Subsystem4 ==
  Step2 : Step  Time=40.17  Before=1  After=0  SampleTime=0
  Trig : Outport
  wires:
  Step2/1 -> Trig/1
